simulink library "Generator_Lib"  (R2019a)
settings: Solver=VariableStepAuto  StartTime=0.0  StopTime=10.0  RelTol=1e-3
undefined symbols (not defined in the file): block_angle, D1, Delta, DiscIntNeverNeededParam, fao, Ts
libraries: powerlib x56, powerlib_extras x9, simulink x8, sps_avr x2, powerlib_meascontrol x2
(part 2 of 2)

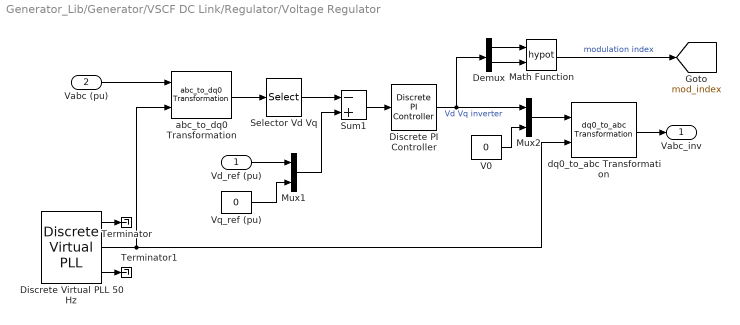
== system Generator_Lib/Generator/VSCF DC Link/Regulator/Voltage Regulator ==
  Vd_ref (pu) : Inport
  Vabc (pu) : Inport  Port=2
  Demux : Demux  Outputs=2
  Discrete PI Controller : powerlib_extras/Discrete  Control Blocks/Discrete PI Controller  Kp=Kp  Ki=Ki  Par_Limits=[1 -1]  Init=0  Ts=Ts
      settings: SourceProductName=Simscape Electrical
  Discrete Virtual PLL 50 Hz : powerlib_extras/Discrete  Control Blocks/Discrete Virtual PLL  Freq=400  Phase=0  Ts=Ts
      settings: SourceProductName=Simscape Electrical  SourceProductBaseCode=PS
  Math Function : Math  Operator=hypot  SaturateOnIntegerOverflow=on
  Mux1 : Mux  Inputs=2
  Mux2 : Mux  Inputs=2
  Selector Vd Vq : Selector  InputPortWidth=3  IndexOptions=Index vector (dialog)  Indices=[1 2]  OutputSizes=1
  Sum1 : Sum  Inputs=-+  SaturateOnIntegerOverflow=on  InputSameDT=on  OutDataTypeStr=Inherit: Same as first input
  Terminator : Terminator
  Terminator1 : Terminator
  V0 : Constant  Value=0
  Vq_ref (pu) : Constant  Value=0
  abc_to_dq0 Transformation : powerlib_extras/Measurements/abc_to_dq0 Transformation
      settings: SourceProductName=Simscape Electrical  SourceProductBaseCode=PS
  dq0_to_abc Transformation : powerlib_extras/Measurements/dq0_to_abc Transformation
      settings: SourceProductName=Simscape Electrical  SourceProductBaseCode=PS
  Vabc_inv : Outport
  tag scope: mod_index=global
  wires:
  Math Function/1 -> [mod_index]  "modulation index"
  Demux/2 -> Math Function/2
  Demux/1 -> Math Function/1
  Discrete PI Controller/1 -> Mux2/1, Demux/1  "Vd Vq inverter"
  Discrete Virtual PLL 50 Hz/3 -> Terminator1/1
  Discrete Virtual PLL 50 Hz/1 -> Terminator/1
  Mux1/1 -> Sum1/2
  Vq_ref (pu)/1 -> Mux1/2
  Vd_ref (pu)/1 -> Mux1/1
  Discrete Virtual PLL 50 Hz/2 -> dq0_to_abc Transformation/2, abc_to_dq0 Transformation/2
  dq0_to_abc Transformation/1 -> Vabc_inv/1
  V0/1 -> Mux2/2
  Mux2/1 -> dq0_to_abc Transformation/1
  Sum1/1 -> Discrete PI Controller/1
  Selector Vd Vq/1 -> Sum1/1
  Vabc (pu)/1 -> abc_to_dq0 Transformation/1
  abc_to_dq0 Transformation/1 -> Selector Vd Vq/1

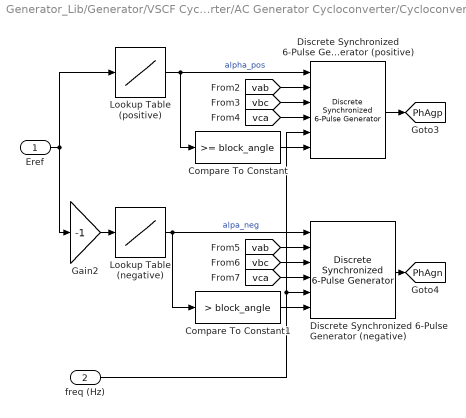
== system Generator_Lib/Generator/VSCF Cycloconverter/AC Generator Cycloconverter/Cycloconverter control (Vsync)/Cyclo Firing Control PhA ==
  Eref : Inport
  freq (Hz) : Inport  Port=2
  Compare To Constant : simulink/Logic and Bit Operations/Compare To Constant  relop=>=  const=block_angle  OutDataTypeStr=boolean  ZeroCross=off
  Compare To Constant1 : simulink/Logic and Bit Operations/Compare To Constant  relop=>  const=block_angle  OutDataTypeStr=boolean  ZeroCross=off
  Discrete Synchronized 6-Pulse Generator (negative) : powerlib_extras/Discrete  Control Blocks/Discrete Synchronized 6-Pulse Generator  pwidth=150  Double_Pulse=off  Ts=Ts
      settings: SourceProductName=Simscape Electrical  SourceProductBaseCode=PS
  Discrete Synchronized 6-Pulse Generator (positive) : powerlib_extras/Discrete  Control Blocks/Discrete Synchronized 6-Pulse Generator  pwidth=150  Double_Pulse=off  Ts=Ts
      settings: SourceProductName=Simscape Electrical  SourceProductBaseCode=PS
  Gain2 : Gain  Gain=-1
  Lookup Table (negative) : Lookup  InputValues=[-1 0 1]  Table=[90 90 0]+fao
  Lookup Table (positive) : Lookup  InputValues=[-1 0 1]  Table=[90 90 0]+fao
  tag scope: PhAgn=global, PhAgp=global
  wires:
  freq (Hz)/1 -> Discrete Synchronized 6-Pulse Generator (negative)/5, Discrete Synchronized 6-Pulse Generator (positive)/5
  Gain2/1 -> Lookup Table (negative)/1
  Compare To Constant1/1 -> Discrete Synchronized 6-Pulse Generator (negative)/6
  Eref/1 -> Gain2/1, Lookup Table (positive)/1
  Lookup Table (negative)/1 -> Compare To Constant1/1, Discrete Synchronized 6-Pulse Generator (negative)/1  "alpa_neg"
  Lookup Table (positive)/1 -> Discrete Synchronized 6-Pulse Generator (positive)/1, Compare To Constant/1  "alpha_pos"
  Compare To Constant/1 -> Discrete Synchronized 6-Pulse Generator (positive)/6
  [vca] -> Discrete Synchronized 6-Pulse Generator (negative)/4
  [vbc] -> Discrete Synchronized 6-Pulse Generator (negative)/3
  [vab] -> Discrete Synchronized 6-Pulse Generator (negative)/2
  [vab] -> Discrete Synchronized 6-Pulse Generator (positive)/2
  [vbc] -> Discrete Synchronized 6-Pulse Generator (positive)/3
  [vca] -> Discrete Synchronized 6-Pulse Generator (positive)/4
  Discrete Synchronized 6-Pulse Generator (negative)/1 -> [PhAgn]
  Discrete Synchronized 6-Pulse Generator (positive)/1 -> [PhAgp]

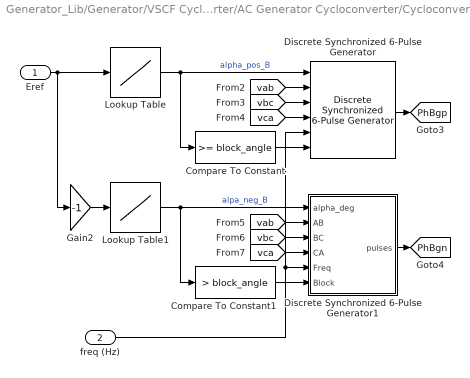
== system Generator_Lib/Generator/VSCF Cycloconverter/AC Generator Cycloconverter/Cycloconverter control (Vsync)/Cyclo Firing Control PhB ==
  Eref : Inport
  freq (Hz) : Inport  Port=2
  Compare To Constant : simulink/Logic and Bit Operations/Compare To Constant  relop=>=  const=block_angle  OutDataTypeStr=boolean  ZeroCross=off
  Compare To Constant1 : simulink/Logic and Bit Operations/Compare To Constant  relop=>  const=block_angle  OutDataTypeStr=boolean  ZeroCross=off
  Discrete Synchronized 6-Pulse Generator : powerlib_extras/Discrete  Control Blocks/Discrete Synchronized 6-Pulse Generator  pwidth=150  Double_Pulse=off  Ts=Ts
      settings: SourceProductName=Simscape Electrical  SourceProductBaseCode=PS
  Discrete Synchronized 6-Pulse Generator1 : Subsystem  DialogController=POWERSYS.PowerSysDialog  mask(Discrete Synchronized 6-pulse generator){pwidth=150, Double_Pulse=off, Ts=Ts}
      mask prompts: pwidth "Pulse width (degrees) :"; Double_Pulse "Double pulsing"; Ts "Time step (s) :"
      mask help:
      | Use this block to fire the 6 thyristors of a 6-pulse converter.
      |
      | The output is a vector of 6 pulses (0-1) individually synchronized on the 6 commutation voltages. Pulses are generated alpha degrees after the increasing zero-crossings of the commutation voltages.
      |
      | Input 1 is  the alpha firing signal (degrees).
      | Inputs 2, 3 and 4 are the synchronization voltages AB BC CA which should be in phase with the 3 phase-phase voltages at the converter terminals.
      | Input 5: Frequency of the synchronization voltages (use a constant or the Freq PLL output)
      | Input 6 allows  blocking of the pulses when the applied signal is non zero.
      |
      | When the 'Douple pulsing' option is checked, two pulses are sent to each thyristor: a 1st pulse when the aplha angle is reached, then a 2nd pulse 60 degrees later, when the next thyristor is fired.
      mask init:
      | power_initmask();
      mask Help: This block is part of a subset of blocks in the Extras library that does not have documentation associated with it, other than the block mask description.
      mask Display: plot(0,0,100,100,[80 62 62 47 47 30],[40 40 60 60 40 40]-5)
  Gain2 : Gain  Gain=-1
  Lookup Table : Lookup  InputValues=[-1 0 1]  Table=[90 90 0]+fao
  Lookup Table1 : Lookup  InputValues=[-1 0 1]  Table=[90 90 0]+fao
  tag scope: PhBgn=global, PhBgp=global
  wires:
  freq (Hz)/1 -> Discrete Synchronized 6-Pulse Generator/5, Discrete Synchronized 6-Pulse Generator1/5(Freq)
  Gain2/1 -> Lookup Table1/1
  Compare To Constant1/1 -> Discrete Synchronized 6-Pulse Generator1/6(Block)
  Discrete Synchronized 6-Pulse Generator/1 -> [PhBgp]
  Discrete Synchronized 6-Pulse Generator1/1(pulses) -> [PhBgn]
  [vca] -> Discrete Synchronized 6-Pulse Generator/4
  [vbc] -> Discrete Synchronized 6-Pulse Generator/3
  [vab] -> Discrete Synchronized 6-Pulse Generator/2
  [vab] -> Discrete Synchronized 6-Pulse Generator1/2(AB)
  [vbc] -> Discrete Synchronized 6-Pulse Generator1/3(BC)
  [vca] -> Discrete Synchronized 6-Pulse Generator1/4(CA)
  Compare To Constant/1 -> Discrete Synchronized 6-Pulse Generator/6
  Lookup Table/1 -> Discrete Synchronized 6-Pulse Generator/1, Compare To Constant/1  "alpha_pos_B"
  Lookup Table1/1 -> Discrete Synchronized 6-Pulse Generator1/1(alpha_deg), Compare To Constant1/1  "alpa_neg_B"
  Eref/1 -> Gain2/1, Lookup Table/1

== system Generator_Lib/Generator/VSCF Cycloconverter/AC Generator Cycloconverter/Cycloconverter control (Vsync)/Cyclo Firing Control PhC ==
  Eref : Inport
  freq (Hz) : Inport  Port=2
  Compare To Constant : simulink/Logic and Bit Operations/Compare To Constant  relop=>=  const=block_angle  OutDataTypeStr=boolean  ZeroCross=off
  Compare To Constant1 : simulink/Logic and Bit Operations/Compare To Constant  relop=>  const=block_angle  OutDataTypeStr=boolean  ZeroCross=off
  Discrete Synchronized 6-Pulse Generator : powerlib_extras/Discrete  Control Blocks/Discrete Synchronized 6-Pulse Generator  pwidth=120  Double_Pulse=off  Ts=Ts
      settings: SourceProductName=Simscape Electrical  SourceProductBaseCode=PS
  Discrete Synchronized 6-Pulse Generator1 : Subsystem  DialogController=POWERSYS.PowerSysDialog  mask(Discrete Synchronized 6-pulse generator){pwidth=120, Double_Pulse=off, Ts=Ts}
      mask prompts: pwidth "Pulse width (degrees) :"; Double_Pulse "Double pulsing"; Ts "Time step (s) :"
      mask help:
      | Use this block to fire the 6 thyristors of a 6-pulse converter.
      |
      | The output is a vector of 6 pulses (0-1) individually synchronized on the 6 commutation voltages. Pulses are generated alpha degrees after the increasing zero-crossings of the commutation voltages.
      |
      | Input 1 is  the alpha firing signal (degrees).
      | Inputs 2, 3 and 4 are the synchronization voltages AB BC CA which should be in phase with the 3 phase-phase voltages at the converter terminals.
      | Input 5: Frequency of the synchronization voltages (use a constant or the Freq PLL output)
      | Input 6 allows  blocking of the pulses when the applied signal is non zero.
      |
      | When the 'Douple pulsing' option is checked, two pulses are sent to each thyristor: a 1st pulse when the aplha angle is reached, then a 2nd pulse 60 degrees later, when the next thyristor is fired.
      mask init:
      | power_initmask();
      mask Help: This block is part of a subset of blocks in the Extras library that does not have documentation associated with it, other than the block mask description.
      mask Display: plot(0,0,100,100,[80 62 62 47 47 30],[40 40 60 60 40 40]-5)
  Gain2 : Gain  Gain=-1
  Lookup Table : Lookup  InputValues=[-1 0 1]  Table=[90 90 0]+fao
  Lookup Table1 : Lookup  InputValues=[-1 0 1]  Table=[90 90 0]+fao
  tag scope: PhCgn=global, PhCgp=global
  wires:
  Gain2/1 -> Lookup Table1/1
  freq (Hz)/1 -> Discrete Synchronized 6-Pulse Generator/5, Discrete Synchronized 6-Pulse Generator1/5(Freq)
  Compare To Constant1/1 -> Discrete Synchronized 6-Pulse Generator1/6(Block)
  Eref/1 -> Gain2/1, Lookup Table/1
  Lookup Table1/1 -> Discrete Synchronized 6-Pulse Generator1/1(alpha_deg), Compare To Constant1/1  "alpa_neg_C"
  Lookup Table/1 -> Discrete Synchronized 6-Pulse Generator/1, Compare To Constant/1  "alpha_pos_C"
  Compare To Constant/1 -> Discrete Synchronized 6-Pulse Generator/6
  [vca] -> Discrete Synchronized 6-Pulse Generator1/4(CA)
  [vbc] -> Discrete Synchronized 6-Pulse Generator1/3(BC)
  [vab] -> Discrete Synchronized 6-Pulse Generator1/2(AB)
  [vab] -> Discrete Synchronized 6-Pulse Generator/2
  [vbc] -> Discrete Synchronized 6-Pulse Generator/3
  [vca] -> Discrete Synchronized 6-Pulse Generator/4
  Discrete Synchronized 6-Pulse Generator1/1(pulses) -> [PhCgn]
  Discrete Synchronized 6-Pulse Generator/1 -> [PhCgp]

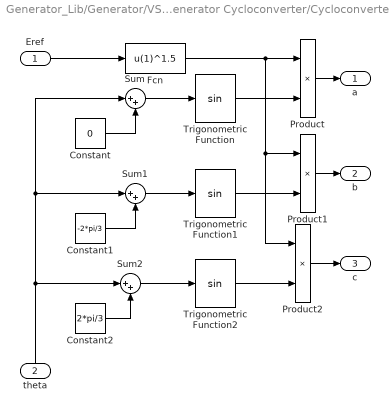
== system Generator_Lib/Generator/VSCF Cycloconverter/AC Generator Cycloconverter/Cycloconverter control (Vsync)/Sine ==
  Eref : Inport
  theta : Inport  Port=2
  Constant : Constant  Value=0
  Constant1 : Constant  Value=-2*pi/3
  Constant2 : Constant  Value=2*pi/3
  Fcn : Fcn  Expr=u(1)^1.5
  Product : Product  RndMeth=Zero
  Product1 : Product  RndMeth=Zero
  Product2 : Product  RndMeth=Zero
  Sum : Sum  Inputs=|++
  Sum1 : Sum  Inputs=|++
  Sum2 : Sum  Inputs=|++
  Trigonometric Function : Trigonometry
  Trigonometric Function1 : Trigonometry
  Trigonometric Function2 : Trigonometry
  a : Outport
  b : Outport  Port=2
  c : Outport  Port=3
  wires:
  Fcn/1 -> Product2/1, Product1/1, Product/1
  Eref/1 -> Fcn/1
  Product2/1 -> c/1
  Product1/1 -> b/1
  Product/1 -> a/1
  Trigonometric Function2/1 -> Product2/2
  Constant2/1 -> Sum2/2
  Sum2/1 -> Trigonometric Function2/1
  Trigonometric Function1/1 -> Product1/2
  Constant1/1 -> Sum1/2
  Sum1/1 -> Trigonometric Function1/1
  Trigonometric Function/1 -> Product/2
  Constant/1 -> Sum/2
  Sum/1 -> Trigonometric Function/1
  theta/1 -> Sum2/1, Sum/1, Sum1/1

== system Generator_Lib/Generator/VSCF Cycloconverter/AC Generator Cycloconverter/Ideal Source/Sensing ==
  Constant : Constant  Value=[1 1]*12000  SampleTime=-1
  Constant1 : Constant  Value=202  SampleTime=-1
  Mux : Mux  Inputs=3
  rpm2pu1 : Gain  Gain=2*pi/60
  tag scope: Gen1Data=global
  wires:
  Constant/1 -> rpm2pu1/1  "Spd"
  Mux/1 -> [Gen1Data]
  rpm2pu1/1 -> Mux/1
  Constant1/1 -> Mux/2
  [Pwr_Gen1_Only] -> Mux/3

== system Generator_Lib/Generator/VSCF DC Link/DC Link Gen/Ideal/Sensing ==
  Constant : Constant  Value=[1 1]*12000  SampleTime=-1
  Constant1 : Constant  Value=202  SampleTime=-1
  Mux : Mux  Inputs=3
  rpm2pu1 : Gain  Gain=2*pi/60
  tag scope: Gen1Data=global
  wires:
  Constant/1 -> rpm2pu1/1  "Spd"
  Mux/1 -> [Gen1Data]
  rpm2pu1/1 -> Mux/1
  Constant1/1 -> Mux/2
  [Pwr_Gen1_Only] -> Mux/3

== system Generator_Lib/Generator/VSCF DC Link/DC Link Gen/Sync Mach/Displays ==
  w : Inport
  Frequency (Hz) : Display
      settings: Decimation=100  SampleTime=1e-2
  Gain : Gain  Gain=30/pi
  Gain3 : Gain  Gain=1/30
  Rate Transition : RateTransition  OutPortSampleTimeOpt=Inherit  OutPortSampleTime=Ts
  Rate Transition1 : RateTransition  OutPortSampleTimeOpt=Inherit  OutPortSampleTime=Ts
  Speed (RPM) : Display
      settings: Decimation=100  SampleTime=1e-2
  wires:
  w/1 -> Gain/1
  Rate Transition/1 -> Speed (RPM)/1
  Gain3/1 -> Rate Transition1/1
  Gain/1 -> Rate Transition/1, Gain3/1
  Rate Transition1/1 -> Frequency (Hz)/1

== system Generator_Lib/Generator/VSCF DC Link/DC Link Gen/Sync Mach/Generator Control Unit (GCU) ==
  Iabc : Inport
  Vabc : Inport  Port=2
  PMG : Inport  Port=3
  Demux : Demux  Outputs=3
  Excitation System : sps_avr/Excitation System  tr=20e-3  reg=[ 300, 0.001 ]  exc=[ 1, 0 ]  tgr=[ 0, 0 ]  damp=[ 0.001, 0.1 ]  sat=[ 0, 0 ]  lim=[ -2, 2, 0 ]  v0=[1 1*203.1/200]
      settings: SourceProductName=Simscape Electrical  SourceProductBaseCode=PS
  Integrator : Integrator
  PU_SI : Gain  Gain=200
  SI_PU : Gain  Gain=1/(200*sqrt(2))
  Terminator1 : Terminator
  Terminator2 : Terminator
  Vref : Constant
  abc to dq0 : powerlib_meascontrol/Transformations/abc to dq0  Alignment=90 degrees behind phase A axis
      settings: SourceProductName=Simscape Electrical
  threshold3 : Constant  Value=0
  V Field : Outport
  tag scope: Gen1_Vfield=global
  wires:
  Vabc/1 -> SI_PU/1
  PMG/1 -> Integrator/1
  Integrator/1 -> abc to dq0/2
  abc to dq0/1 -> Demux/1
  Demux/1 -> Excitation System/2
  Demux/2 -> Excitation System/3
  SI_PU/1 -> abc to dq0/1
  Excitation System/1 -> PU_SI/1
  PU_SI/1 -> V Field/1, [Gen1_Vfield]
  Vref/1 -> Excitation System/1
  threshold3/1 -> Excitation System/4
  Iabc/1 -> Terminator1/1
  Demux/3 -> Terminator2/1

== system Generator_Lib/Generator/VSCF DC Link/DC Link Gen/Sync Mach/Generator Control Breaker (GCB) ==
  GLC : Inport
  Close switch : Subsystem
  Complex to Real-Imag : ComplexToRealImag  Output=Real
  Complex to Real-Imag1 : ComplexToRealImag  Output=Real
  Contactor : Subsystem
  Memory : Memory
  P.O.R  and CTA : powerlib/Measurements/Three-Phase V-I Measurement  VoltageMeasurement=phase-to-phase  SetLabelV=off  LabelV=Vabc_Gen1  Vpu=off  VpuLL=off  CurrentMeasurement=yes  SetLabelI=off  LabelI=Iabc_Gen1  Ipu=off  Pbase=100e6  Vbase=500e3  OutputType=Complex  PhasorSimulation=off  PSBequivalent=0
      settings: SourceProductName=Simscape Electrical
  in_a : PMIOPort  Side=Left
  in_b : PMIOPort  Port=2  Side=Left
  in_c : PMIOPort  Port=3  Side=Left
  out_a : PMIOPort  Port=4  Side=Right
  out_b : PMIOPort  Port=5  Side=Right
  out_c : PMIOPort  Port=6  Side=Right
  Vabc : Outport
  Iabc : Outport  Port=2
  wires:
  Close switch/1(Out1) -> Contactor/1(com)
  Memory/1 -> Close switch/1(In1)
  Complex to Real-Imag1/1 -> Iabc/1
  Complex to Real-Imag/1 -> Vabc/1
  P.O.R  and CTA/2 -> Complex to Real-Imag1/1
  P.O.R  and CTA/1 -> Complex to Real-Imag/1
  GLC/1 -> Memory/1
  connections:
  Contactor/RConn3 -- out_c/RConn1
  Contactor/RConn1 -- out_a/RConn1
  P.O.R  and CTA/RConn2 -- Contactor/LConn2
  Contactor/LConn3 -- P.O.R  and CTA/RConn3
  P.O.R  and CTA/LConn3 -- in_c/RConn1
  in_b/RConn1 -- P.O.R  and CTA/LConn2
  P.O.R  and CTA/LConn1 -- in_a/RConn1
  Contactor/LConn1 -- P.O.R  and CTA/RConn1
  out_b/RConn1 -- Contactor/RConn2

== system Generator_Lib/Generator/VSCF DC Link/DC Link Gen/Sync Mach/Sensing ==
  In1 : Inport
  Data : Subsystem
  Mux : Mux  Inputs=3
  tag scope: Gen1Data=global
  wires:
  Mux/1 -> [Gen1Data]
  In1/1 -> Data/1(B)
  Data/1(w) -> Mux/1
  Data/2(Vf) -> Mux/2
  Data/3(Pe) -> Mux/3

== system Generator_Lib/Generator/VSCF DC Link/DC Link Gen/Sync Mach/Vab ==
  Voltage Measurement : powerlib/Measurements/Voltage Measurement  PhasorSimulation=off  OutputType=Magnitude  PSBequivalent=0
      settings: SourceProductName=Simscape Electrical
  + : PMIOPort  Side=Right
  - : PMIOPort  Port=2  Side=Right
  tag scope: Gen1_Vab=global
  wires:
  Voltage Measurement/1 -> [Gen1_Vab]
  connections:
  Voltage Measurement/LConn2 -- -/RConn1
  Voltage Measurement/LConn1 -- +/RConn1

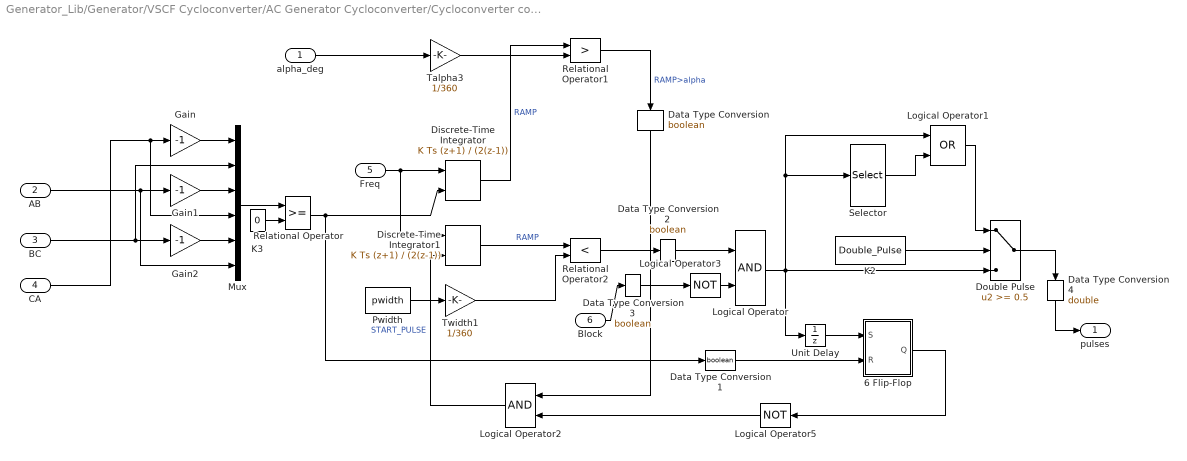
== system Generator_Lib/Generator/VSCF Cycloconverter/AC Generator Cycloconverter/Cycloconverter control (Vsync)/Cyclo Firing Control PhB/Discrete Synchronized 6-Pulse Generator1 ==
  alpha_deg : Inport
  AB : Inport  Port=2
  BC : Inport  Port=3
  CA : Inport  Port=4
  Freq : Inport  Port=5
  Block : Inport  Port=6
  6 Flip-Flop : Subsystem
  Data Type Conversion{,1..3} (4 alike) : DataTypeConversion  OutDataTypeStr=boolean  SaturateOnIntegerOverflow=on  RndMeth=Zero
  Data Type Conversion4 : DataTypeConversion  OutDataTypeStr=double  SaturateOnIntegerOverflow=on  RndMeth=Zero
  Discrete-Time Integrator : DiscreteIntegrator  IntegratorMethod=Integration: Trapezoidal  ExternalReset=rising  SampleTime=Ts  ICPrevOutput=DiscIntNeverNeededParam  ICPrevScaledInput=DiscIntNeverNeededParam
  Discrete-Time Integrator1 : DiscreteIntegrator  IntegratorMethod=Integration: Trapezoidal  ExternalReset=rising  SampleTime=Ts  ICPrevOutput=DiscIntNeverNeededParam  ICPrevScaledInput=DiscIntNeverNeededParam
  Double Pulse : Switch  Threshold=0.5  InputSameDT=on
  Gain : Gain  Gain=-1  SaturateOnIntegerOverflow=on  OutDataTypeStr=Inherit: Same as input  ParamDataTypeStr=Inherit: Same as input
  Gain1 : Gain  Gain=-1  SaturateOnIntegerOverflow=on  OutDataTypeStr=Inherit: Same as input  ParamDataTypeStr=Inherit: Same as input
  Gain2 : Gain  Gain=-1  SaturateOnIntegerOverflow=on  OutDataTypeStr=Inherit: Same as input  ParamDataTypeStr=Inherit: Same as input
  K2 : Constant  Value=Double_Pulse
  K3 : Constant  Value=0
  Logical Operator : Logic
  Logical Operator1 : Logic  Operator=OR
  Logical Operator2 : Logic
  Logical Operator3 : Logic  Operator=NOT  Inputs=1
  Logical Operator5 : Logic  Operator=NOT  Inputs=1
  Mux : Mux  Inputs=6
  Pwidth : Constant  Value=pwidth
  Relational Operator : RelationalOperator  RndMeth=Nearest  InputSameDT=on
  Relational Operator1 : RelationalOperator  Operator=>  RndMeth=Nearest  InputSameDT=on
  Relational Operator2 : RelationalOperator  Operator=<  RndMeth=Nearest  InputSameDT=on
  Selector : Selector  InputPortWidth=6  IndexOptions=Index vector (dialog)  Indices=[2 3 4 5 6 1 ]  OutputSizes=1
  Talpha3 : Gain  Gain=1/360  SaturateOnIntegerOverflow=on  OutDataTypeStr=Inherit: Same as input  ParamDataTypeStr=Inherit: Same as input
  Twidth1 : Gain  Gain=1/360  SaturateOnIntegerOverflow=on  OutDataTypeStr=Inherit: Same as input  ParamDataTypeStr=Inherit: Same as input
  Unit Delay : UnitDelay  SampleTime=Ts  HasFrameUpgradeWarning=on
  pulses : Outport  InitialOutput=0
  wires:
  Data Type Conversion4/1 -> pulses/1
  Double Pulse/1 -> Data Type Conversion4/1
  Data Type Conversion3/1 -> Logical Operator3/1
  Block/1 -> Data Type Conversion3/1
  Data Type Conversion2/1 -> Logical Operator/1
  Relational Operator2/1 -> Data Type Conversion2/1
  Data Type Conversion1/1 -> 6 Flip-Flop/2(R)
  Data Type Conversion/1 -> Logical Operator2/1
  Relational Operator1/1 -> Data Type Conversion/1  "RAMP>alpha"
  Logical Operator2/1 -> Discrete-Time Integrator1/2  "START_PULSE"
  AB/1 -> Mux/6, Gain1/1
  Logical Operator3/1 -> Logical Operator/2
  Unit Delay/1 -> 6 Flip-Flop/1(S)
  K2/1 -> Double Pulse/2
  Logical Operator/1 -> Unit Delay/1, Double Pulse/3, Selector/1, Logical Operator1/1
  Selector/1 -> Logical Operator1/2
  Logical Operator1/1 -> Double Pulse/1
  Pwidth/1 -> Twidth1/1
  Twidth1/1 -> Relational Operator2/2
  Discrete-Time Integrator1/1 -> Relational Operator2/1  "RAMP"
  Discrete-Time Integrator/1 -> Relational Operator1/1  "RAMP"
  Gain/1 -> Mux/1
  Gain1/1 -> Mux/3
  Gain2/1 -> Mux/5
  K3/1 -> Relational Operator/2
  Relational Operator/1 -> Data Type Conversion1/1, Discrete-Time Integrator/2
  Logical Operator5/1 -> Logical Operator2/2
  Talpha3/1 -> Relational Operator1/2
  Mux/1 -> Relational Operator/1
  CA/1 -> Gain/1, Mux/4
  BC/1 -> Gain2/1, Mux/2
  Freq/1 -> Discrete-Time Integrator/1, Discrete-Time Integrator1/1
  6 Flip-Flop/1(Q) -> Logical Operator5/1
  alpha_deg/1 -> Talpha3/1

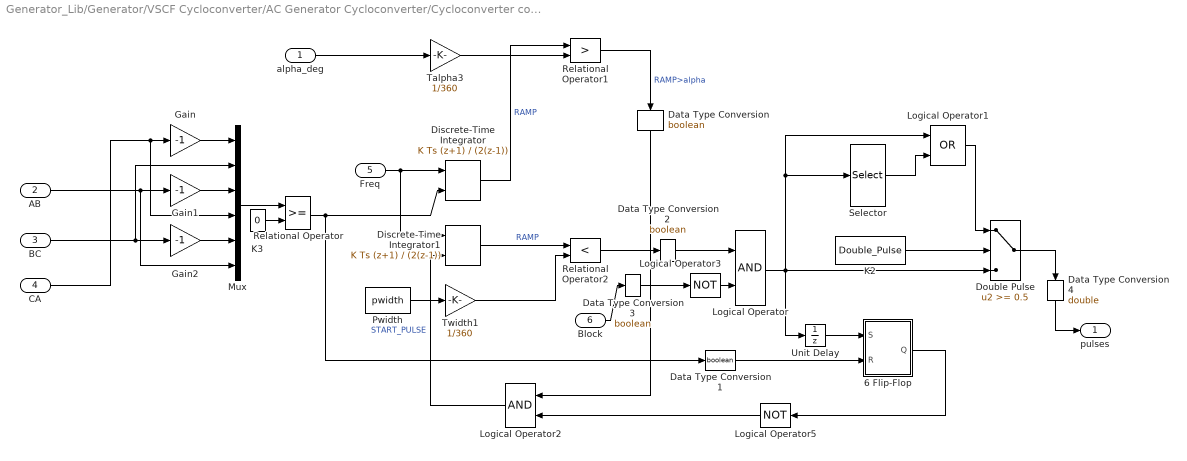
== system Generator_Lib/Generator/VSCF Cycloconverter/AC Generator Cycloconverter/Cycloconverter control (Vsync)/Cyclo Firing Control PhC/Discrete Synchronized 6-Pulse Generator1 ==
  alpha_deg : Inport
  AB : Inport  Port=2
  BC : Inport  Port=3
  CA : Inport  Port=4
  Freq : Inport  Port=5
  Block : Inport  Port=6
  6 Flip-Flop : Subsystem
  Data Type Conversion{,1..3} (4 alike) : DataTypeConversion  OutDataTypeStr=boolean  SaturateOnIntegerOverflow=on  RndMeth=Zero
  Data Type Conversion4 : DataTypeConversion  OutDataTypeStr=double  SaturateOnIntegerOverflow=on  RndMeth=Zero
  Discrete-Time Integrator : DiscreteIntegrator  IntegratorMethod=Integration: Trapezoidal  ExternalReset=rising  SampleTime=Ts  ICPrevOutput=DiscIntNeverNeededParam  ICPrevScaledInput=DiscIntNeverNeededParam
  Discrete-Time Integrator1 : DiscreteIntegrator  IntegratorMethod=Integration: Trapezoidal  ExternalReset=rising  SampleTime=Ts  ICPrevOutput=DiscIntNeverNeededParam  ICPrevScaledInput=DiscIntNeverNeededParam
  Double Pulse : Switch  Threshold=0.5  InputSameDT=on
  Gain : Gain  Gain=-1  SaturateOnIntegerOverflow=on  OutDataTypeStr=Inherit: Same as input  ParamDataTypeStr=Inherit: Same as input
  Gain1 : Gain  Gain=-1  SaturateOnIntegerOverflow=on  OutDataTypeStr=Inherit: Same as input  ParamDataTypeStr=Inherit: Same as input
  Gain2 : Gain  Gain=-1  SaturateOnIntegerOverflow=on  OutDataTypeStr=Inherit: Same as input  ParamDataTypeStr=Inherit: Same as input
  K2 : Constant  Value=Double_Pulse
  K3 : Constant  Value=0
  Logical Operator : Logic
  Logical Operator1 : Logic  Operator=OR
  Logical Operator2 : Logic
  Logical Operator3 : Logic  Operator=NOT  Inputs=1
  Logical Operator5 : Logic  Operator=NOT  Inputs=1
  Mux : Mux  Inputs=6
  Pwidth : Constant  Value=pwidth
  Relational Operator : RelationalOperator  RndMeth=Nearest  InputSameDT=on
  Relational Operator1 : RelationalOperator  Operator=>  RndMeth=Nearest  InputSameDT=on
  Relational Operator2 : RelationalOperator  Operator=<  RndMeth=Nearest  InputSameDT=on
  Selector : Selector  InputPortWidth=6  IndexOptions=Index vector (dialog)  Indices=[2 3 4 5 6 1 ]  OutputSizes=1
  Talpha3 : Gain  Gain=1/360  SaturateOnIntegerOverflow=on  OutDataTypeStr=Inherit: Same as input  ParamDataTypeStr=Inherit: Same as input
  Twidth1 : Gain  Gain=1/360  SaturateOnIntegerOverflow=on  OutDataTypeStr=Inherit: Same as input  ParamDataTypeStr=Inherit: Same as input
  Unit Delay : UnitDelay  SampleTime=Ts  HasFrameUpgradeWarning=on
  pulses : Outport  InitialOutput=0
  wires:
  Data Type Conversion4/1 -> pulses/1
  Double Pulse/1 -> Data Type Conversion4/1
  Data Type Conversion3/1 -> Logical Operator3/1
  Block/1 -> Data Type Conversion3/1
  Data Type Conversion2/1 -> Logical Operator/1
  Relational Operator2/1 -> Data Type Conversion2/1
  Data Type Conversion1/1 -> 6 Flip-Flop/2(R)
  Data Type Conversion/1 -> Logical Operator2/1
  Relational Operator1/1 -> Data Type Conversion/1  "RAMP>alpha"
  Logical Operator2/1 -> Discrete-Time Integrator1/2  "START_PULSE"
  AB/1 -> Mux/6, Gain1/1
  Logical Operator3/1 -> Logical Operator/2
  Unit Delay/1 -> 6 Flip-Flop/1(S)
  K2/1 -> Double Pulse/2
  Logical Operator/1 -> Unit Delay/1, Double Pulse/3, Selector/1, Logical Operator1/1
  Selector/1 -> Logical Operator1/2
  Logical Operator1/1 -> Double Pulse/1
  Pwidth/1 -> Twidth1/1
  Twidth1/1 -> Relational Operator2/2
  Discrete-Time Integrator1/1 -> Relational Operator2/1  "RAMP"
  Discrete-Time Integrator/1 -> Relational Operator1/1  "RAMP"
  Gain/1 -> Mux/1
  Gain1/1 -> Mux/3
  Gain2/1 -> Mux/5
  K3/1 -> Relational Operator/2
  Relational Operator/1 -> Data Type Conversion1/1, Discrete-Time Integrator/2
  Logical Operator5/1 -> Logical Operator2/2
  Talpha3/1 -> Relational Operator1/2
  Mux/1 -> Relational Operator/1
  CA/1 -> Gain/1, Mux/4
  BC/1 -> Gain2/1, Mux/2
  Freq/1 -> Discrete-Time Integrator/1, Discrete-Time Integrator1/1
  6 Flip-Flop/1(Q) -> Logical Operator5/1
  alpha_deg/1 -> Talpha3/1

== system Generator_Lib/Generator/VSCF DC Link/DC Link Gen/Sync Mach/Generator Control Breaker (GCB)/Close switch ==
  In1 : Inport
  Data Type Conversion : DataTypeConversion
  Rad_Rpm : Gain  Gain=30/pi
  Relay : Relay  OnSwitchValue=9000  OffSwitchValue=8900
  Out1 : Outport
  wires:
  In1/1 -> Rad_Rpm/1
  Relay/1 -> Data Type Conversion/1
  Rad_Rpm/1 -> Relay/1
  Data Type Conversion/1 -> Out1/1

== system Generator_Lib/Generator/VSCF DC Link/DC Link Gen/Sync Mach/Generator Control Breaker (GCB)/Contactor ==
  com : Inport
  Three-Phase Breaker : powerlib/Elements/Three-Phase Breaker  InitialState=open  SwitchA=on  SwitchB=on  SwitchC=on  SwitchTimes="[4/60  10/60]"  External=on  BreakerResistance=0.001  SnubberResistance=1e3  SnubberCapacitance=inf  Measurements=None
      settings: SourceProductName=Simscape Electrical
  A : PMIOPort  Side=Left
  a : PMIOPort  Port=2  Side=Right
  B : PMIOPort  Port=3  Side=Left
  b : PMIOPort  Port=4  Side=Right
  C : PMIOPort  Port=5  Side=Left
  c : PMIOPort  Port=6  Side=Right
  wires:
  com/1 -> Three-Phase Breaker/1
  connections:
  C/RConn1 -- Three-Phase Breaker/LConn3
  B/RConn1 -- Three-Phase Breaker/LConn2
  A/RConn1 -- Three-Phase Breaker/LConn1
  c/RConn1 -- Three-Phase Breaker/RConn3
  Three-Phase Breaker/RConn2 -- b/RConn1
  a/RConn1 -- Three-Phase Breaker/RConn1

== system Generator_Lib/Generator/VSCF DC Link/DC Link Gen/Sync Mach/Sensing/Data ==
  B : Inport
  Bus Selector : BusSelector  OutputSignals=Rotor speed wm (rad/s),Electrical power Pe (W),Terminal voltage Va (V),Terminal voltage Vb (V),Terminal voltage Vc (V),Stator current is_a (A),Stator current is_b (A),Stator current is_c (A)
  Constant : Constant  Value=12000
  Mux : Mux  Inputs=2
  Mux1 : Mux  Inputs=3
  Mux2 : Mux  Inputs=3
  rpm2pu1 : Gain  Gain=2*pi/60
  w : Outport
  Vf : Outport  Port=2
  Pe : Outport  Port=3
  tag scope: Iabc_Gen1Only=global, Vabc_Gen1Only=global
  wires:
  [Gen1_Vfield] -> Vf/1
  B/1 -> Bus Selector/1
  Bus Selector/2 -> Pe/1  "<Electrical power Pe (W)>"
  Bus Selector/1 -> Mux/1  "<Rotor speed wm (rad/s)>"
  rpm2pu1/1 -> Mux/2
  Constant/1 -> rpm2pu1/1  "Spd"
  Mux/1 -> w/1
  Bus Selector/3 -> Mux1/1  "<Terminal voltage Va (V)>"
  Bus Selector/4 -> Mux1/2  "<Terminal voltage Vb (V)>"
  Bus Selector/5 -> Mux1/3  "<Terminal voltage Vc (V)>"
  Mux1/1 -> [Vabc_Gen1Only]
  Mux2/1 -> [Iabc_Gen1Only]
  Bus Selector/6 -> Mux2/1  "<Stator current is_a (A)>"
  Bus Selector/7 -> Mux2/2  "<Stator current is_b (A)>"
  Bus Selector/8 -> Mux2/3  "<Stator current is_c (A)>"

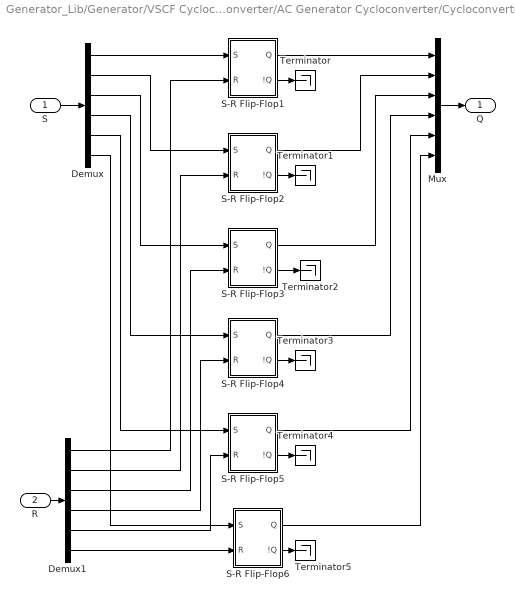
== system Generator_Lib/Generator/VSCF Cycloconverter/AC Generator Cycloconverter/Cycloconverter control (Vsync)/Cyclo Firing Control PhB/Discrete Synchronized 6-Pulse Generator1/6 Flip-Flop ==
  S : Inport
  R : Inport  Port=2
  Demux : Demux  Outputs=6
  Demux1 : Demux  Outputs=6
  Mux : Mux  Inputs=6
  S-R Flip-Flop1 : Subsystem  mask(SRFlipFlop){initial_condition=0, Ts=Ts}
      mask prompts: initial_condition "Initial condition:"; Ts "Sample time:"
      mask help: S-R Flip Flop Block
  S-R Flip-Flop2 : Subsystem  mask(SRFlipFlop){initial_condition=0, Ts=Ts}
      mask prompts: initial_condition "Initial condition:"; Ts "Sample time:"
      mask help: S-R Flip Flop Block
  S-R Flip-Flop3 : Subsystem  mask(SRFlipFlop){initial_condition=0, Ts=Ts}
      mask prompts: initial_condition "Initial condition:"; Ts "Sample time:"
      mask help: S-R Flip Flop Block
  S-R Flip-Flop4 : Subsystem  mask(SRFlipFlop){initial_condition=0, Ts=Ts}
      mask prompts: initial_condition "Initial condition:"; Ts "Sample time:"
      mask help: S-R Flip Flop Block
  S-R Flip-Flop5 : Subsystem  mask(SRFlipFlop){initial_condition=0, Ts=Ts}
      mask prompts: initial_condition "Initial condition:"; Ts "Sample time:"
      mask help: S-R Flip Flop Block
  S-R Flip-Flop6 : Subsystem  mask(SRFlipFlop){initial_condition=0, Ts=Ts}
      mask prompts: initial_condition "Initial condition:"; Ts "Sample time:"
      mask help: S-R Flip Flop Block
  Terminator{,1..5} (6 alike) : Terminator
  Q : Outport
  wires:
  S-R Flip-Flop6/2(!Q) -> Terminator5/1
  S-R Flip-Flop5/2(!Q) -> Terminator4/1
  S-R Flip-Flop4/2(!Q) -> Terminator3/1
  S-R Flip-Flop3/2(!Q) -> Terminator2/1
  S-R Flip-Flop2/2(!Q) -> Terminator1/1
  S-R Flip-Flop1/1(Q) -> Mux/1
  S-R Flip-Flop2/1(Q) -> Mux/2
  S-R Flip-Flop3/1(Q) -> Mux/3
  S-R Flip-Flop4/1(Q) -> Mux/4
  S-R Flip-Flop5/1(Q) -> Mux/5
  Mux/1 -> Q/1
  S-R Flip-Flop6/1(Q) -> Mux/6
  S-R Flip-Flop1/2(!Q) -> Terminator/1
  Demux/1 -> S-R Flip-Flop1/1(S)
  Demux/2 -> S-R Flip-Flop2/1(S)
  Demux/3 -> S-R Flip-Flop3/1(S)
  Demux/4 -> S-R Flip-Flop4/1(S)
  S/1 -> Demux/1
  Demux/6 -> S-R Flip-Flop6/1(S)
  Demux/5 -> S-R Flip-Flop5/1(S)
  R/1 -> Demux1/1
  Demux1/1 -> S-R Flip-Flop1/2(R)
  Demux1/2 -> S-R Flip-Flop2/2(R)
  Demux1/3 -> S-R Flip-Flop3/2(R)
  Demux1/4 -> S-R Flip-Flop4/2(R)
  Demux1/5 -> S-R Flip-Flop5/2(R)
  Demux1/6 -> S-R Flip-Flop6/2(R)

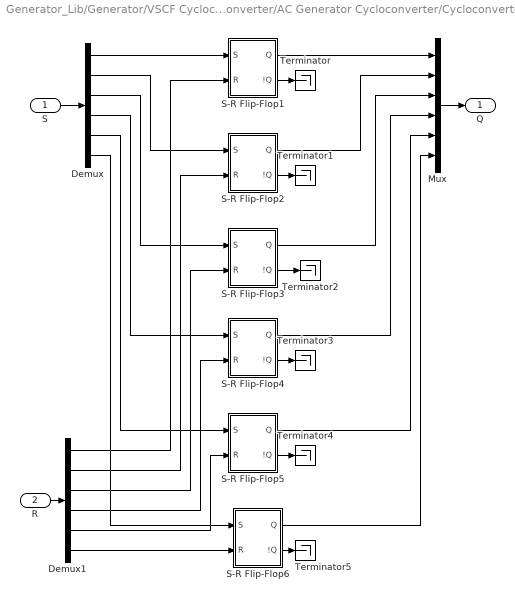
== system Generator_Lib/Generator/VSCF Cycloconverter/AC Generator Cycloconverter/Cycloconverter control (Vsync)/Cyclo Firing Control PhC/Discrete Synchronized 6-Pulse Generator1/6 Flip-Flop ==
  S : Inport
  R : Inport  Port=2
  Demux : Demux  Outputs=6
  Demux1 : Demux  Outputs=6
  Mux : Mux  Inputs=6
  S-R Flip-Flop1 : Subsystem  mask(SRFlipFlop){initial_condition=0, Ts=Ts}
      mask prompts: initial_condition "Initial condition:"; Ts "Sample time:"
      mask help: S-R Flip Flop Block
  S-R Flip-Flop2 : Subsystem  mask(SRFlipFlop){initial_condition=0, Ts=Ts}
      mask prompts: initial_condition "Initial condition:"; Ts "Sample time:"
      mask help: S-R Flip Flop Block
  S-R Flip-Flop3 : Subsystem  mask(SRFlipFlop){initial_condition=0, Ts=Ts}
      mask prompts: initial_condition "Initial condition:"; Ts "Sample time:"
      mask help: S-R Flip Flop Block
  S-R Flip-Flop4 : Subsystem  mask(SRFlipFlop){initial_condition=0, Ts=Ts}
      mask prompts: initial_condition "Initial condition:"; Ts "Sample time:"
      mask help: S-R Flip Flop Block
  S-R Flip-Flop5 : Subsystem  mask(SRFlipFlop){initial_condition=0, Ts=Ts}
      mask prompts: initial_condition "Initial condition:"; Ts "Sample time:"
      mask help: S-R Flip Flop Block
  S-R Flip-Flop6 : Subsystem  mask(SRFlipFlop){initial_condition=0, Ts=Ts}
      mask prompts: initial_condition "Initial condition:"; Ts "Sample time:"
      mask help: S-R Flip Flop Block
  Terminator{,1..5} (6 alike) : Terminator
  Q : Outport
  wires:
  S-R Flip-Flop6/2(!Q) -> Terminator5/1
  S-R Flip-Flop5/2(!Q) -> Terminator4/1
  S-R Flip-Flop4/2(!Q) -> Terminator3/1
  S-R Flip-Flop3/2(!Q) -> Terminator2/1
  S-R Flip-Flop2/2(!Q) -> Terminator1/1
  S-R Flip-Flop1/1(Q) -> Mux/1
  S-R Flip-Flop2/1(Q) -> Mux/2
  S-R Flip-Flop3/1(Q) -> Mux/3
  S-R Flip-Flop4/1(Q) -> Mux/4
  S-R Flip-Flop5/1(Q) -> Mux/5
  Mux/1 -> Q/1
  S-R Flip-Flop6/1(Q) -> Mux/6
  S-R Flip-Flop1/2(!Q) -> Terminator/1
  Demux/1 -> S-R Flip-Flop1/1(S)
  Demux/2 -> S-R Flip-Flop2/1(S)
  Demux/3 -> S-R Flip-Flop3/1(S)
  Demux/4 -> S-R Flip-Flop4/1(S)
  S/1 -> Demux/1
  Demux/6 -> S-R Flip-Flop6/1(S)
  Demux/5 -> S-R Flip-Flop5/1(S)
  R/1 -> Demux1/1
  Demux1/1 -> S-R Flip-Flop1/2(R)
  Demux1/2 -> S-R Flip-Flop2/2(R)
  Demux1/3 -> S-R Flip-Flop3/2(R)
  Demux1/4 -> S-R Flip-Flop4/2(R)
  Demux1/5 -> S-R Flip-Flop5/2(R)
  Demux1/6 -> S-R Flip-Flop6/2(R)

== system Generator_Lib/Generator/VSCF Cycloconverter/AC Generator Cycloconverter/Cycloconverter control (Vsync)/Cyclo Firing Control PhB/Discrete Synchronized 6-Pulse Generator1/6 Flip-Flop/S-R Flip-Flop1 ==
  S : Inport
  R : Inport  Port=2
  Demux : Demux  Outputs=2
  Logic : CombinatorialLogic  TruthTable=[0 1;0 1;1 0;0 1;1 0;0 1;1 0;1 0]
  Mux : Mux  Inputs=3
  Unit Delay : UnitDelay  InitialCondition=initial_condition  SampleTime=Ts  HasFrameUpgradeWarning=on
  Q : Outport  InitialOutput=0
  !Q : Outport  Port=2  InitialOutput=1
  wires:
  R/1 -> Mux/3
  S/1 -> Mux/2
  Unit Delay/1 -> Mux/1
  Demux/1 -> Unit Delay/1, Q/1
  Demux/2 -> !Q/1
  Logic/1 -> Demux/1
  Mux/1 -> Logic/1

== system Generator_Lib/Generator/VSCF Cycloconverter/AC Generator Cycloconverter/Cycloconverter control (Vsync)/Cyclo Firing Control PhB/Discrete Synchronized 6-Pulse Generator1/6 Flip-Flop/S-R Flip-Flop2 ==
  S : Inport
  R : Inport  Port=2
  Demux : Demux  Outputs=2
  Logic : CombinatorialLogic  TruthTable=[0 1;0 1;1 0;0 1;1 0;0 1;1 0;1 0]
  Mux : Mux  Inputs=3
  Unit Delay : UnitDelay  InitialCondition=initial_condition  SampleTime=Ts  HasFrameUpgradeWarning=on
  Q : Outport  InitialOutput=0
  !Q : Outport  Port=2  InitialOutput=1
  wires:
  Mux/1 -> Logic/1
  Logic/1 -> Demux/1
  Demux/2 -> !Q/1
  Demux/1 -> Q/1, Unit Delay/1
  Unit Delay/1 -> Mux/1
  S/1 -> Mux/2
  R/1 -> Mux/3

== system Generator_Lib/Generator/VSCF Cycloconverter/AC Generator Cycloconverter/Cycloconverter control (Vsync)/Cyclo Firing Control PhB/Discrete Synchronized 6-Pulse Generator1/6 Flip-Flop/S-R Flip-Flop3 ==
  S : Inport
  R : Inport  Port=2
  Demux : Demux  Outputs=2
  Logic : CombinatorialLogic  TruthTable=[0 1;0 1;1 0;0 1;1 0;0 1;1 0;1 0]
  Mux : Mux  Inputs=3
  Unit Delay : UnitDelay  InitialCondition=initial_condition  SampleTime=Ts  HasFrameUpgradeWarning=on
  Q : Outport  InitialOutput=0
  !Q : Outport  Port=2  InitialOutput=1
  wires:
  R/1 -> Mux/3
  S/1 -> Mux/2
  Unit Delay/1 -> Mux/1
  Demux/1 -> Unit Delay/1, Q/1
  Demux/2 -> !Q/1
  Logic/1 -> Demux/1
  Mux/1 -> Logic/1

== system Generator_Lib/Generator/VSCF Cycloconverter/AC Generator Cycloconverter/Cycloconverter control (Vsync)/Cyclo Firing Control PhB/Discrete Synchronized 6-Pulse Generator1/6 Flip-Flop/S-R Flip-Flop4 ==
  S : Inport
  R : Inport  Port=2
  Demux : Demux  Outputs=2
  Logic : CombinatorialLogic  TruthTable=[0 1;0 1;1 0;0 1;1 0;0 1;1 0;1 0]
  Mux : Mux  Inputs=3
  Unit Delay : UnitDelay  InitialCondition=initial_condition  SampleTime=Ts  HasFrameUpgradeWarning=on
  Q : Outport  InitialOutput=0
  !Q : Outport  Port=2  InitialOutput=1
  wires:
  Mux/1 -> Logic/1
  Logic/1 -> Demux/1
  Demux/2 -> !Q/1
  Demux/1 -> Q/1, Unit Delay/1
  Unit Delay/1 -> Mux/1
  S/1 -> Mux/2
  R/1 -> Mux/3

== system Generator_Lib/Generator/VSCF Cycloconverter/AC Generator Cycloconverter/Cycloconverter control (Vsync)/Cyclo Firing Control PhB/Discrete Synchronized 6-Pulse Generator1/6 Flip-Flop/S-R Flip-Flop5 ==
  S : Inport
  R : Inport  Port=2
  Demux : Demux  Outputs=2
  Logic : CombinatorialLogic  TruthTable=[0 1;0 1;1 0;0 1;1 0;0 1;1 0;1 0]
  Mux : Mux  Inputs=3
  Unit Delay : UnitDelay  InitialCondition=initial_condition  SampleTime=Ts  HasFrameUpgradeWarning=on
  Q : Outport  InitialOutput=0
  !Q : Outport  Port=2  InitialOutput=1
  wires:
  R/1 -> Mux/3
  S/1 -> Mux/2
  Unit Delay/1 -> Mux/1
  Demux/1 -> Unit Delay/1, Q/1
  Demux/2 -> !Q/1
  Logic/1 -> Demux/1
  Mux/1 -> Logic/1

== system Generator_Lib/Generator/VSCF Cycloconverter/AC Generator Cycloconverter/Cycloconverter control (Vsync)/Cyclo Firing Control PhB/Discrete Synchronized 6-Pulse Generator1/6 Flip-Flop/S-R Flip-Flop6 ==
  S : Inport
  R : Inport  Port=2
  Demux : Demux  Outputs=2
  Logic : CombinatorialLogic  TruthTable=[0 1;0 1;1 0;0 1;1 0;0 1;1 0;1 0]
  Mux : Mux  Inputs=3
  Unit Delay : UnitDelay  InitialCondition=initial_condition  SampleTime=Ts  HasFrameUpgradeWarning=on
  Q : Outport  InitialOutput=0
  !Q : Outport  Port=2  InitialOutput=1
  wires:
  Mux/1 -> Logic/1
  Logic/1 -> Demux/1
  Demux/2 -> !Q/1
  Demux/1 -> Q/1, Unit Delay/1
  Unit Delay/1 -> Mux/1
  S/1 -> Mux/2
  R/1 -> Mux/3

== system Generator_Lib/Generator/VSCF Cycloconverter/AC Generator Cycloconverter/Cycloconverter control (Vsync)/Cyclo Firing Control PhC/Discrete Synchronized 6-Pulse Generator1/6 Flip-Flop/S-R Flip-Flop1 ==
  S : Inport
  R : Inport  Port=2
  Demux : Demux  Outputs=2
  Logic : CombinatorialLogic  TruthTable=[0 1;0 1;1 0;0 1;1 0;0 1;1 0;1 0]
  Mux : Mux  Inputs=3
  Unit Delay : UnitDelay  InitialCondition=initial_condition  SampleTime=Ts  HasFrameUpgradeWarning=on
  Q : Outport  InitialOutput=0
  !Q : Outport  Port=2  InitialOutput=1
  wires:
  R/1 -> Mux/3
  S/1 -> Mux/2
  Unit Delay/1 -> Mux/1
  Demux/1 -> Unit Delay/1, Q/1
  Demux/2 -> !Q/1
  Logic/1 -> Demux/1
  Mux/1 -> Logic/1

== system Generator_Lib/Generator/VSCF Cycloconverter/AC Generator Cycloconverter/Cycloconverter control (Vsync)/Cyclo Firing Control PhC/Discrete Synchronized 6-Pulse Generator1/6 Flip-Flop/S-R Flip-Flop2 ==
  S : Inport
  R : Inport  Port=2
  Demux : Demux  Outputs=2
  Logic : CombinatorialLogic  TruthTable=[0 1;0 1;1 0;0 1;1 0;0 1;1 0;1 0]
  Mux : Mux  Inputs=3
  Unit Delay : UnitDelay  InitialCondition=initial_condition  SampleTime=Ts  HasFrameUpgradeWarning=on
  Q : Outport  InitialOutput=0
  !Q : Outport  Port=2  InitialOutput=1
  wires:
  Mux/1 -> Logic/1
  Logic/1 -> Demux/1
  Demux/2 -> !Q/1
  Demux/1 -> Q/1, Unit Delay/1
  Unit Delay/1 -> Mux/1
  S/1 -> Mux/2
  R/1 -> Mux/3

== system Generator_Lib/Generator/VSCF Cycloconverter/AC Generator Cycloconverter/Cycloconverter control (Vsync)/Cyclo Firing Control PhC/Discrete Synchronized 6-Pulse Generator1/6 Flip-Flop/S-R Flip-Flop3 ==
  S : Inport
  R : Inport  Port=2
  Demux : Demux  Outputs=2
  Logic : CombinatorialLogic  TruthTable=[0 1;0 1;1 0;0 1;1 0;0 1;1 0;1 0]
  Mux : Mux  Inputs=3
  Unit Delay : UnitDelay  InitialCondition=initial_condition  SampleTime=Ts  HasFrameUpgradeWarning=on
  Q : Outport  InitialOutput=0
  !Q : Outport  Port=2  InitialOutput=1
  wires:
  R/1 -> Mux/3
  S/1 -> Mux/2
  Unit Delay/1 -> Mux/1
  Demux/1 -> Unit Delay/1, Q/1
  Demux/2 -> !Q/1
  Logic/1 -> Demux/1
  Mux/1 -> Logic/1

== system Generator_Lib/Generator/VSCF Cycloconverter/AC Generator Cycloconverter/Cycloconverter control (Vsync)/Cyclo Firing Control PhC/Discrete Synchronized 6-Pulse Generator1/6 Flip-Flop/S-R Flip-Flop4 ==
  S : Inport
  R : Inport  Port=2
  Demux : Demux  Outputs=2
  Logic : CombinatorialLogic  TruthTable=[0 1;0 1;1 0;0 1;1 0;0 1;1 0;1 0]
  Mux : Mux  Inputs=3
  Unit Delay : UnitDelay  InitialCondition=initial_condition  SampleTime=Ts  HasFrameUpgradeWarning=on
  Q : Outport  InitialOutput=0
  !Q : Outport  Port=2  InitialOutput=1
  wires:
  Mux/1 -> Logic/1
  Logic/1 -> Demux/1
  Demux/2 -> !Q/1
  Demux/1 -> Q/1, Unit Delay/1
  Unit Delay/1 -> Mux/1
  S/1 -> Mux/2
  R/1 -> Mux/3

== system Generator_Lib/Generator/VSCF Cycloconverter/AC Generator Cycloconverter/Cycloconverter control (Vsync)/Cyclo Firing Control PhC/Discrete Synchronized 6-Pulse Generator1/6 Flip-Flop/S-R Flip-Flop5 ==
  S : Inport
  R : Inport  Port=2
  Demux : Demux  Outputs=2
  Logic : CombinatorialLogic  TruthTable=[0 1;0 1;1 0;0 1;1 0;0 1;1 0;1 0]
  Mux : Mux  Inputs=3
  Unit Delay : UnitDelay  InitialCondition=initial_condition  SampleTime=Ts  HasFrameUpgradeWarning=on
  Q : Outport  InitialOutput=0
  !Q : Outport  Port=2  InitialOutput=1
  wires:
  R/1 -> Mux/3
  S/1 -> Mux/2
  Unit Delay/1 -> Mux/1
  Demux/1 -> Unit Delay/1, Q/1
  Demux/2 -> !Q/1
  Logic/1 -> Demux/1
  Mux/1 -> Logic/1

== system Generator_Lib/Generator/VSCF Cycloconverter/AC Generator Cycloconverter/Cycloconverter control (Vsync)/Cyclo Firing Control PhC/Discrete Synchronized 6-Pulse Generator1/6 Flip-Flop/S-R Flip-Flop6 ==
  S : Inport
  R : Inport  Port=2
  Demux : Demux  Outputs=2
  Logic : CombinatorialLogic  TruthTable=[0 1;0 1;1 0;0 1;1 0;0 1;1 0;1 0]
  Mux : Mux  Inputs=3
  Unit Delay : UnitDelay  InitialCondition=initial_condition  SampleTime=Ts  HasFrameUpgradeWarning=on
  Q : Outport  InitialOutput=0
  !Q : Outport  Port=2  InitialOutput=1
  wires:
  Mux/1 -> Logic/1
  Logic/1 -> Demux/1
  Demux/2 -> !Q/1
  Demux/1 -> Q/1, Unit Delay/1
  Unit Delay/1 -> Mux/1
  S/1 -> Mux/2
  R/1 -> Mux/3
